simulink model "filter_IIR3"  (Simulink 7.9)
settings: Solver=ode3  StartTime=0.0  StopTime=0.08  FixedStep=0.125e-3  RelTol=1e-3
libraries: simulink x1
settings Model: Creator=asus  LastModifiedBy=asus  BufferReuse=off
settings OptimizationCC: OptimizeBlockIOStorage=off  BufferReuse=off  ExpressionFolding=off  LocalBlockOutputs=off

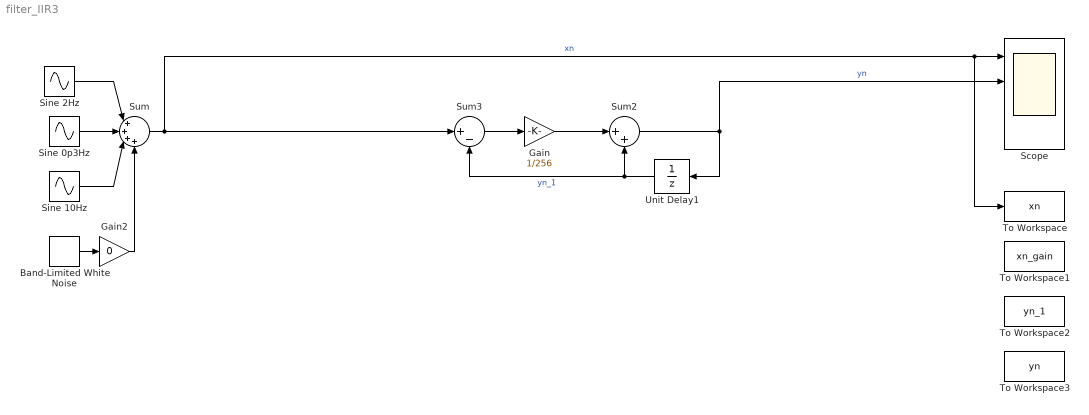
== system filter_IIR3 ==
  Band-Limited White Noise : simulink/Sources/Band-Limited White Noise  Cov=[1.25e-7]  Ts=0.125e-3  seed=[23341]
  Gain : Gain  Gain=1/256  OutDataTypeStr=int32
  Gain2 : Gain  Gain=0
  Scope : Scope  NumInputPorts=4
      settings: ShowLegends=on  TimeRange=20  YMin=0.98~-2~-2.5~-5  YMax=1.04~2~2.5~5  MaxDataPoints=65536  SampleInput=on  SampleTime=0.125e-3
  Sine 0p3Hz : Sin  Amplitude=0  Frequency=0.3*2*pi  SampleTime=0.125e-3
  Sine 10Hz : Sin  Amplitude=0  Frequency=10*2*pi  SampleTime=0.125e-3
  Sine 2Hz : Sin  Amplitude=1*1024  Bias=1024  Frequency=0*2*pi  SampleTime=0.125e-3
  Sum : Sum  Inputs=|++++  OutDataTypeStr=int32  SampleTime=0.125e-3
  Sum2 : Sum  Inputs=|++  OutDataTypeStr=int32  SampleTime=0.125e-3
  Sum3 : Sum  Inputs=|+-  OutDataTypeStr=int32  SampleTime=0.125e-3
  To Workspace : ToWorkspace  VariableName=xn  SampleTime=0.125e-3  SaveFormat=Timeseries
  To Workspace1 : ToWorkspace  VariableName=xn_gain  SampleTime=0.125e-3  SaveFormat=Timeseries
  To Workspace2 : ToWorkspace  VariableName=yn_1  SampleTime=0.125e-3  SaveFormat=Timeseries
  To Workspace3 : ToWorkspace  VariableName=yn  SampleTime=0.125e-3  SaveFormat=Timeseries
  Unit Delay1 : UnitDelay  SampleTime=0.125e-3
  wires:
  Sine 2Hz/1 -> Sum/1
  Sum/1 -> Scope/1, To Workspace/1, Sum3/1  "xn"
  Sine 0p3Hz/1 -> Sum/2
  Sine 10Hz/1 -> Sum/3
  Band-Limited White Noise/1 -> Gain2/1
  Gain2/1 -> Sum/4
  Sum2/1 -> Unit Delay1/1, Scope/2  "yn"
  Unit Delay1/1 -> Sum2/2, Sum3/2  "yn_1"
  Sum3/1 -> Gain/1
  Gain/1 -> Sum2/1
